simulink subsystem "Trajectory"  (R2020a)
settings: Solver=VariableStepAuto  StartTime=0.0  StopTime=10.0  RelTol=1e-3
undefined symbols (not defined in the file): initposearray
libraries: robotlib x3, vxlib1 x1
settings Model: Creator=Lamarre  LastModifiedBy=lamarre

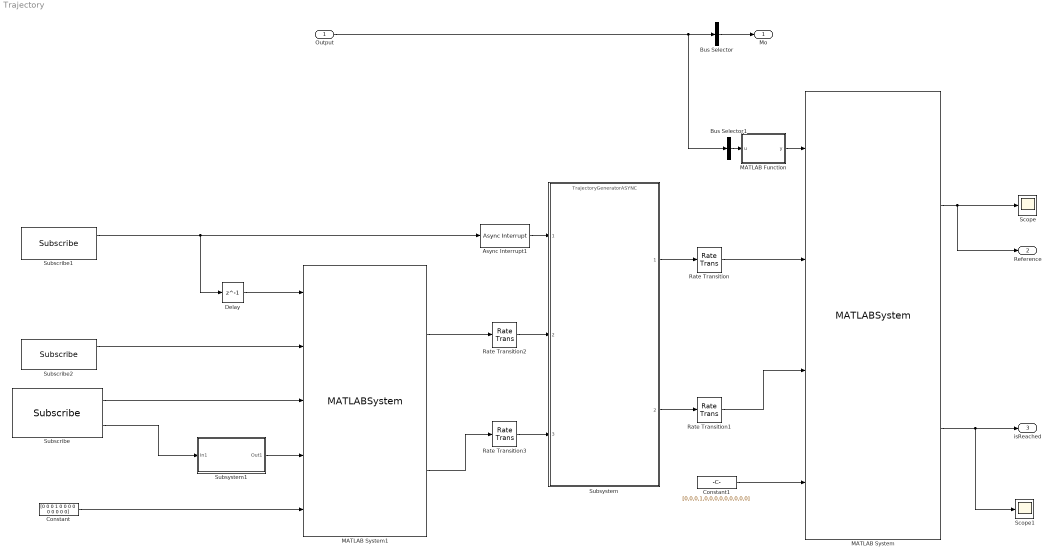
== system Trajectory ==
  Output : Inport
  Async Interrupt1 : vxlib1/Async Interrupt  irqnumbers=[1 ]  irqoffsets=[192 ]  irqpriorities=[10 ]  irqpreempts=[0 ]  manageowntimer=on  tickres=1/60  ticklen=32bits  showinput=on
      settings: SourceProductBaseCode=SL
  Bus Selector : BusSelector  OutputSignals=World Position,qS2W,Body Velocity,Angular Rate,Roll;Pitch; Yaw  OutputAsBus=on
  Bus Selector1 : BusSelector  OutputSignals=World Position,qS2W  OutputAsBus=on
  Constant : Constant  Value=[0 0 0 1 0 0 0 0 0 0 0 0 0]  VectorParams1D=off
  Constant1 : Constant  Value=[0,0,0,1,0,0,0,0,0,0,0,0,0]
  Delay : Delay  DelayLength=1
  MATLAB Function : MATLAB Function  TreatAsAtomicUnit=on
  MATLAB System : MATLABSystem  System=TrajectoryManager  SampleTime=.25  OffsetTime=0.2  prediction=4  bufferSize=6001  linearConvergence=.2  quaternionConvergence=.1  TargetThreshold=3  SimulateUsing=Interpreted execution
      mask Type: TrajectoryManager
      mask Display:
      | disp('TrajectoryManager');
      | port_label('input',1,'mesuredPose');
      | port_label('input',2,'poses');
      | port_label('input',3,'isNew');
      | port_label('input',4,'InitCond');
      | port_label('output',1,'currentPose');
      | port_label('output',2,'isReached');
  MATLAB System1 : MATLABSystem  System=AddPose  buffSize=20  elementSize=8  SimulateUsing=Code generation
      mask Type: AddPose
      mask Display:
      | disp('AddPose');
      | port_label('input',1,'compute');
      | port_label('input',2,'clearBuffer');
      | port_label('input',3,'isNew');
      | port_label('input',4,'waypoint');
      | port_label('input',5,'initCond');
      | port_label('output',1,'waypoints');
      | port_label('output',2,'count');
  Rate Transition : RateTransition  Deterministic=off
  Rate Transition1 : RateTransition  Deterministic=off
  Rate Transition2 : RateTransition  Deterministic=off  InitialCondition=initposearray
  Rate Transition3 : RateTransition  Deterministic=off  InitialCondition=2
  Scope : Scope
  Scope1 : Scope
  Subscribe : robotlib/Subscribe  topicSource=Specify your own  topic=proc_control_matlab/add_pose  messageType=sonia_common/AddPose  sampleTime=-1  messageQueueLength=1
      link override SourceBlock: ROSTopic=/my_topic  ROSMessageType=geometry_msgs/Point  SLBusName=SL_Bus_Test_Traj_geometry_msgs_Point  ModelName=Test_Traj  BlockId=Sub_Test_Traj_124
  Subscribe1 : robotlib/Subscribe  topicSource=Specify your own  topic=/proc_control_matlab/compute_trajectory  messageType=std_msgs/Bool  sampleTime=-1  messageQueueLength=1
  Subscribe2 : robotlib/Subscribe  topicSource=Specify your own  topic=/proc_control_matlab/clear_waypoints  messageType=std_msgs/Bool  sampleTime=-1  messageQueueLength=1
  Subsystem : ModelReference  ModelNameDialog=TrajectoryGeneratorASYNC  SimulationMode=Normal  ModelReferenceVersion=1.537
  Subsystem1 : Subsystem
  Mo : Outport
  Reference : Outport  Port=2
  isReached : Outport  Port=3
  wires:
  Output/1 -> Bus Selector/1, Bus Selector1/1
  Bus Selector/1 -> Mo/1
  MATLAB System1/2 -> Rate Transition3/1
  MATLAB System1/1 -> Rate Transition2/1
  MATLAB System/1 -> Scope/1, Reference/1
  Delay/1 -> MATLAB System1/1
  Constant/1 -> MATLAB System1/5
  Constant1/1 -> MATLAB System/4
  Subsystem/1 -> Rate Transition/1
  Rate Transition2/1 -> Subsystem/2
  Rate Transition3/1 -> Subsystem/3
  Subsystem/2 -> Rate Transition1/1
  Subscribe1/1 -> Async Interrupt1/1, Delay/1
  Subsystem1/1(Out1) -> MATLAB System1/4
  Async Interrupt1/1 -> Subsystem/1
  Subscribe/1 -> MATLAB System1/3
  Subscribe/2 -> Subsystem1/1(In1)
  Subscribe2/1 -> MATLAB System1/2
  MATLAB System/2 -> isReached/1, Scope1/1
  Bus Selector1/1 -> MATLAB Function/1(u)
  MATLAB Function/1(y) -> MATLAB System/1
  Rate Transition1/1 -> MATLAB System/3
  Rate Transition/1 -> MATLAB System/2

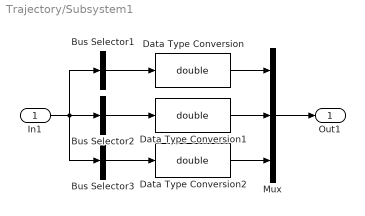
== system Trajectory/Subsystem1 ==
  In1 : Inport
  Bus Selector1 : BusSelector  OutputSignals=Position.X,Position.Y,Position.Z,Orientation.Z,Orientation.Y,Orientation.X  OutputAsBus=on
  Bus Selector2 : BusSelector  OutputSignals=Frame,Speed  OutputAsBus=on
  Bus Selector3 : BusSelector  OutputSignals=Fine  OutputAsBus=on
  Data Type Conversion : DataTypeConversion  OutDataTypeStr=double  LockScale=on
  Data Type Conversion1 : DataTypeConversion  OutDataTypeStr=double  LockScale=on
  Data Type Conversion2 : DataTypeConversion  OutDataTypeStr=double  LockScale=on
  Mux : Mux  Inputs=3
  Out1 : Outport
  wires:
  Mux/1 -> Out1/1
  Data Type Conversion2/1 -> Mux/3
  Data Type Conversion1/1 -> Mux/2
  Data Type Conversion/1 -> Mux/1
  Bus Selector3/1 -> Data Type Conversion2/1
  Bus Selector2/1 -> Data Type Conversion1/1
  In1/1 -> Bus Selector2/1, Bus Selector3/1, Bus Selector1/1
  Bus Selector1/1 -> Data Type Conversion/1

== matlab function Trajectory/MATLAB Function ==
  data: u input size=[1,7]; y output size=[1,7]
function y = fcn(u)

y = u;
